simulink model "sampleModel1962_4"  (R2023a)
settings: Solver=VariableStepAuto  StartTime=0.0  StopTime=10.0  RelTol=1e-3
libraries: hdlsllib x4, simulink x3
settings Model: Creator=user1  LastModifiedBy=user1

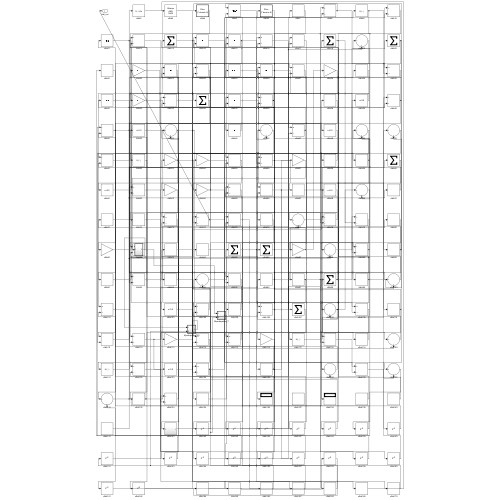
[thumbnail: Simulink's stored preview of the top-level diagram]
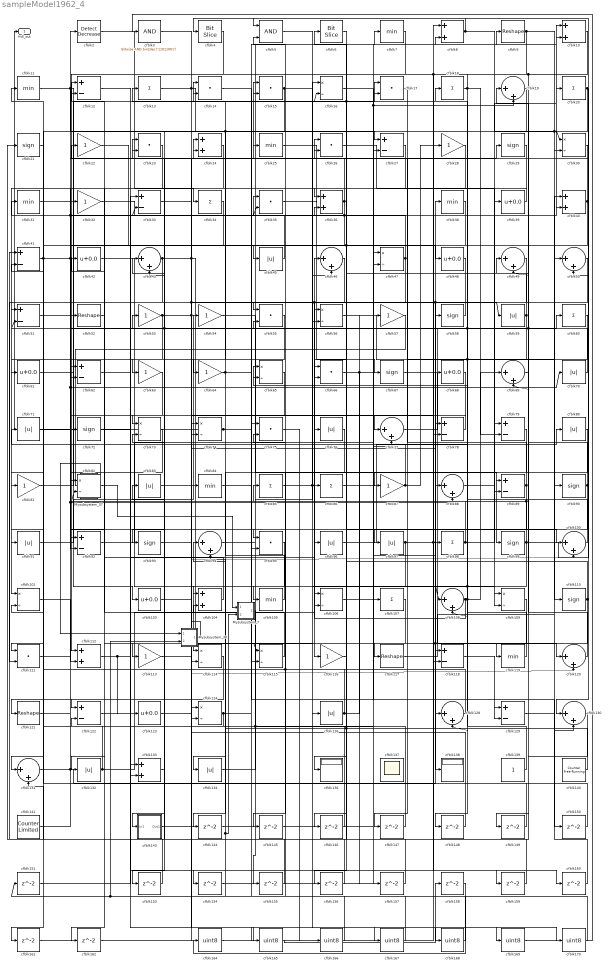
== system sampleModel1962_4 ==
  Mysubsystem_30 : Subsystem  TreatAsAtomicUnit=on  RTWFcnName=Mysubsystem_30
      settings: RTWFcnNameOpts=User specified  RTWFileNameOpts=Use function name
  Mysubsystem_37 : Subsystem  TreatAsAtomicUnit=on  RTWFcnName=Mysubsystem_37
      settings: RTWFcnNameOpts=User specified  RTWFileNameOpts=Use function name
  Mysubsystem_7 : Subsystem  TreatAsAtomicUnit=on  RTWFcnName=Mysubsystem_7
      settings: RTWFcnNameOpts=User specified  RTWFileNameOpts=Use function name
  cfblk{8,10,24,36,40,104,112,133} (8 alike) : Sum  OutDataTypeStr=uint8
  cfblk{19,43,46,49..50,69,77,88,94,100,108,120,128,130..131} (15 alike) : Sum  Inputs=|++  OutDataTypeStr=uint8
  cfblk{16,30,47,56,65,73..74,82,101,106,109,114..115,124} (14 alike) : Product  Inputs=*/  OutDataTypeStr=uint8  RndMeth=Zero  SaturateOnIntegerOverflow=on
  cfblk{39,42,48,61,68,103,123} (7 alike) : Bias  Bias=0.0  SaturateOnIntegerOverflow=off
  cfblk{7,11,25,31,38,84,105,119} (8 alike) : MinMax  OutDataTypeStr=uint8
  cfblk{13,18,20,34,60,85..86,98,107} (9 alike) : Sum  Inputs=+  OutDataTypeStr=uint8
  cfblk{21,29,58,67,72,90,93,99,110} (9 alike) : Signum
  cfblk{14..15,17,23,26,35,55,66,75,95,111} (11 alike) : DotProduct  OutDataTypeStr=uint8
  cfblk{22,28,32,53..54,57,63..64,81,87,113,116} (12 alike) : Gain  OutDataTypeStr=uint8
  cfblk{9,52,117,121} (4 alike) : Reshape
  cfblk{12,27,33,41,51,62,78..79,89,92,118,122,129} (13 alike) : Sum  Inputs=+-  OutDataTypeStr=uint8
  cfblk{45,59,70..71,76,80,83,91,96..97,126,132,134} (13 alike) : Abs  OutDataTypeStr=uint8  SaturateOnIntegerOverflow=off
  cfblk136 : Display
  cfblk137 : Scope
      settings: Floating=on
  cfblk138 : Display
  cfblk139 : Constant  OutDataTypeStr=uint8  SampleTime=-1
  cfblk140 : hdlsllib/Sources/Counter Free-Running  NumBits=16  tsamp=-1
  cfblk141 : hdlsllib/Sources/Counter Limited  uplimit=7  tsamp=-1
  cfblk143 : Subsystem
      settings: LibrarySourceBlock=|
      | hdlsllib/Ports &
      | Subsystems/Subsystem
  cfblk{144..151,153..162} (18 alike) : Delay  SampleTime=1
  cfblk{164..170} (7 alike) : DataTypeConversion  OutDataTypeStr=uint8  SaturateOnIntegerOverflow=off  RndMeth=Floor
  cfblk2 : simulink/Logic and Bit Operations/Detect Decrease  vinit=0.0  OutDataTypeStr=uint8
      settings: LibrarySourceBlock=|
      | hdlsllib/Logic and Bit
      | Operations/Detect
      | Decrease
  cfblk3 : simulink/Logic and Bit Operations/Bitwise Operator  logicop=AND  UseBitMask=on  BitMask=bin2dec('11011001')  BitMaskRealWorld=Stored Integer
      settings: LibrarySourceBlock=|
      | hdlsllib/Logic and Bit
      | Operations/Bitwise
      | Operator
  cfblk4 : hdlsllib/Logic and Bit Operations/Bit Slice  lidx=7  ridx=0
  cfblk5 : Logic  AllPortsSameDT=off  OutDataTypeStr=boolean
  cfblk6 : hdlsllib/Logic and Bit Operations/Bit Slice  lidx=7  ridx=0
  Hdl_out : Outport  OutDataTypeStr=uint8
  wires:
  cfblk134/1 -> cfblk7/1, cfblk27/2
  cfblk11/1 -> cfblk103/1, cfblk27/1
  cfblk131/1 -> cfblk38/1, cfblk55/2
  cfblk90/1 -> cfblk50/2, cfblk19/1, cfblk146/1
  cfblk42/1 -> cfblk114/1
  cfblk81/1 -> cfblk17/1
  cfblk2/1 -> cfblk34/1
  cfblk16/1 -> cfblk107/1, cfblk19/2
  cfblk98/1 -> cfblk85/1, cfblk20/1
  cfblk17/1 -> cfblk77/1
  cfblk22/1 -> cfblk45/1
  cfblk49/1 -> cfblk116/1, cfblk143/1(In1)
  cfblk50/1 -> cfblk138/1, cfblk147/1
  cfblk63/1 -> cfblk112/1
  cfblk78/1 -> cfblk73/1
  cfblk24/1 -> cfblk101/1
  cfblk4/1 -> cfblk72/1
  cfblk58/1 -> cfblk51/1
  cfblk54/1 -> cfblk99/1
  cfblk26/1 -> cfblk109/1
  cfblk64/1 -> cfblk24/1, cfblk130/2
  cfblk67/1 -> cfblk119/1
  cfblk41/1 -> cfblk48/1, cfblk95/2, cfblk131/1
  cfblk96/1 -> cfblk80/1
  cfblk38/1 -> cfblk81/1, cfblk106/1
  cfblk87/1 -> cfblk14/1, cfblk28/1
  cfblk86/1 -> cfblk89/1
  cfblk25/1 -> cfblk67/1
  cfblk45/1 -> cfblk24/2
  cfblk39/1 -> cfblk32/1
  cfblk6/1 -> cfblk136/1
  cfblk108/1 -> cfblk18/1, cfblk69/1, cfblk106/2
  cfblk84/1 -> cfblk9/1
  cfblk48/1 -> cfblk111/1
  cfblk70/1 -> cfblk12/1, cfblk43/1, cfblk49/2
  cfblk119/1 -> cfblk13/1, cfblk51/2
  cfblk92/1 -> cfblk10/1
  cfblk97/1 -> cfblk120/1, cfblk159/1, cfblk105/1
  cfblk43/1 -> cfblk126/1, cfblk78/2, cfblk111/2
  cfblk100/1 -> cfblk71/1
  cfblk115/1 -> cfblk12/2
  cfblk21/1 -> cfblk91/1
  cfblk113/1 -> cfblk29/1
  cfblk99/1 -> cfblk4/1, cfblk134/1, cfblk65/1
  cfblk61/1 -> cfblk10/2
  cfblk40/1 -> cfblk22/1, cfblk43/2
  cfblk71/1 -> cfblk62/1
  cfblk51/1 -> cfblk2/1
  cfblk83/1 -> cfblk54/1
  cfblk132/1 -> cfblk46/1, cfblk41/2
  cfblk27/1 -> cfblk62/2
  cfblk52/1 -> cfblk132/1
  cfblk74/1 -> cfblk56/1, Hdl_out/1
  cfblk139/1 -> cfblk15/1
  cfblk20/1 -> cfblk64/1, cfblk61/1, cfblk130/1
  cfblk23/1 -> cfblk52/1
  cfblk9/1 -> cfblk110/1, cfblk88/1
  cfblk106/1 -> cfblk98/1
  cfblk101/1 -> cfblk112/2
  cfblk118/1 -> cfblk129/1
  cfblk47/1 -> cfblk93/1, cfblk35/1
  cfblk18/1 -> cfblk58/1, cfblk79/2
  cfblk109/1 -> cfblk122/1
  cfblk94/1 -> cfblk16/1
  cfblk89/1 -> cfblk97/1, cfblk82/2, cfblk25/1
  cfblk53/1 -> cfblk55/1, cfblk120/2, cfblk161/1
  cfblk111/1 -> cfblk26/1, cfblk88/2
  cfblk13/1 -> cfblk47/1, cfblk56/2
  cfblk46/1 -> cfblk113/1
  cfblk121/1 -> cfblk53/1
  cfblk143/1(Out1) -> cfblk47/2
  cfblk59/1 -> cfblk108/1, cfblk128/2, cfblk31/1
  cfblk133/1 -> cfblk23/1
  cfblk32/1 -> cfblk40/2
  cfblk130/1 -> cfblk21/1
  cfblk3/1 -> cfblk170/1
  cfblk29/1 -> cfblk76/1
  cfblk104/1 -> cfblk42/1
  cfblk91/1 -> cfblk84/1
  cfblk12/1 -> cfblk100/1
  cfblk36/1 -> cfblk92/2, cfblk33/2, cfblk15/2
  cfblk60/1 -> cfblk117/1, cfblk108/2
  cfblk75/1 -> cfblk166/1
  cfblk14/1 -> cfblk129/2
  cfblk85/1 -> cfblk86/1, cfblk109/2
  cfblk15/1 -> cfblk46/2, cfblk153/1
  cfblk140/1 -> cfblk16/2, cfblk6/1, cfblk104/2
  cfblk112/1 -> cfblk96/1, cfblk123/1
  cfblk30/1 -> cfblk26/2
  cfblk110/1 -> cfblk115/1, cfblk118/1, cfblk66/2
  cfblk93/1 -> cfblk115/2
  cfblk141/1 -> cfblk60/1, cfblk70/1
  cfblk68/1 -> cfblk87/1
  cfblk95/1 -> cfblk104/1
  cfblk55/1 -> cfblk63/1
  cfblk128/1 -> cfblk11/1
  cfblk66/1 -> cfblk128/1, cfblk157/1
  cfblk120/1 -> cfblk49/1
  cfblk107/1 -> cfblk133/2
  cfblk77/1 -> cfblk39/1
  cfblk10/1 -> cfblk74/2, cfblk118/2, cfblk69/2
  cfblk105/1 -> cfblk14/2
  cfblk35/1 -> cfblk68/1
  cfblk34/1 -> cfblk82/1
  cfblk28/1 -> cfblk66/1
  cfblk33/1 -> cfblk100/2, cfblk59/1
  cfblk8/1 -> cfblk30/1, cfblk30/2, cfblk5/1
  cfblk88/1 -> cfblk79/1
  cfblk114/1 -> cfblk121/1
  cfblk79/1 -> cfblk89/2
  cfblk117/1 -> cfblk50/1
  cfblk123/1 -> cfblk78/1
  cfblk56/1 -> cfblk90/1
  cfblk126/1 -> cfblk83/1, cfblk65/2, cfblk57/1
  cfblk124/1 -> cfblk8/2, cfblk122/2
  cfblk7/1 -> cfblk36/1
  cfblk73/1 -> cfblk92/1
  cfblk31/1 -> cfblk95/1, cfblk35/2
  cfblk76/1 -> cfblk144/1
  cfblk144/1 -> cfblk94/2
  cfblk80/1 -> cfblk145/1
  cfblk145/1 -> cfblk77/2
  cfblk146/1 -> cfblk124/1
  cfblk147/1 -> cfblk73/2
  cfblk19/1 -> cfblk148/1
  cfblk148/1 -> cfblk74/1
  cfblk69/1 -> cfblk149/1
  cfblk149/1 -> cfblk101/2
  cfblk129/1 -> cfblk150/1
  cfblk150/1 -> cfblk5/2
  cfblk151/1 -> cfblk133/1
  cfblk153/1 -> cfblk41/1
  cfblk62/1 -> cfblk154/1
  cfblk154/1 -> cfblk17/2
  cfblk155/1 -> cfblk33/1
  cfblk116/1 -> cfblk156/1
  cfblk156/1 -> cfblk131/2
  cfblk157/1 -> cfblk23/2
  cfblk159/1 -> cfblk36/2
  cfblk122/1 -> cfblk160/1
  cfblk160/1 -> cfblk40/1
  cfblk161/1 -> cfblk114/2
  cfblk65/1 -> cfblk162/1
  cfblk162/1 -> cfblk8/1
  cfblk158/1 -> cfblk164/1
  cfblk103/1 -> cfblk165/1
  cfblk165/1 -> cfblk158/1
  cfblk166/1 -> Mysubsystem_7/2(In2), cfblk94/1
  cfblk5/1 -> cfblk167/1
  cfblk167/1 -> cfblk75/1
  cfblk164/1 -> cfblk168/1
  cfblk168/1 -> cfblk75/2
  cfblk72/1 -> cfblk169/1
  cfblk169/1 -> cfblk3/1
  cfblk170/1 -> cfblk151/1, Mysubsystem_30/2(In2)
  cfblk82/1 -> Mysubsystem_7/1(In1)
  Mysubsystem_7/1(Out1) -> cfblk155/1
  Mysubsystem_30/1(Out1) -> cfblk124/2
  cfblk57/1 -> Mysubsystem_37/1(In1)
  Mysubsystem_37/1(Y) -> Mysubsystem_30/1(In1)

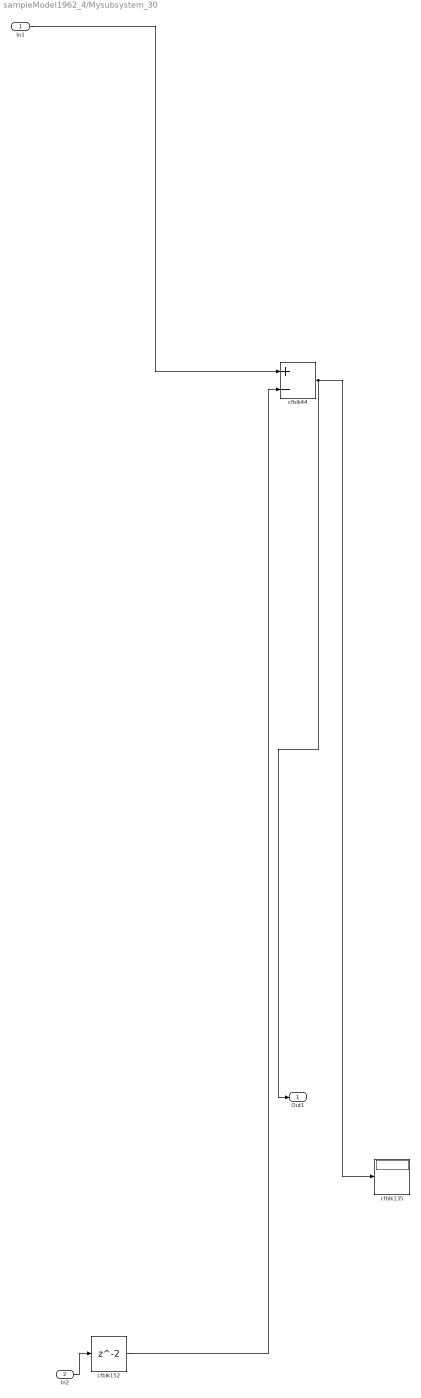
== system sampleModel1962_4/Mysubsystem_30 ==
  In1 : Inport
  In2 : Inport  Port=2
  cfblk135 : Display
  cfblk152 : Delay  SampleTime=1
  cfblk44 : Sum  Inputs=+-
  Out1 : Outport
  wires:
  In1/1 -> cfblk44/1
  cfblk152/1 -> cfblk44/2
  In2/1 -> cfblk152/1
  cfblk44/1 -> Out1/1, cfblk135/1

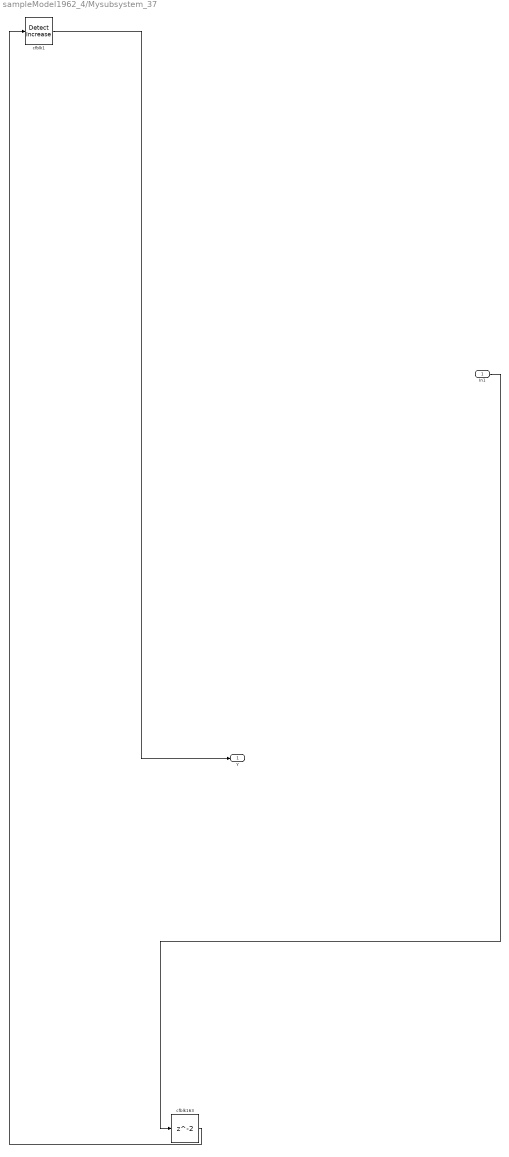
== system sampleModel1962_4/Mysubsystem_37 ==
  In1 : Inport
  cfblk1 : simulink/Logic and Bit Operations/Detect Increase  vinit=0.0  OutDataTypeStr=boolean
      settings: LibrarySourceBlock=|
      | hdlsllib/Logic and Bit
      | Operations/Detect
      | Increase
  cfblk163 : Delay  SampleTime=1
  Y : Outport
  wires:
  cfblk163/1 -> cfblk1/1
  In1/1 -> cfblk163/1
  cfblk1/1 -> Y/1

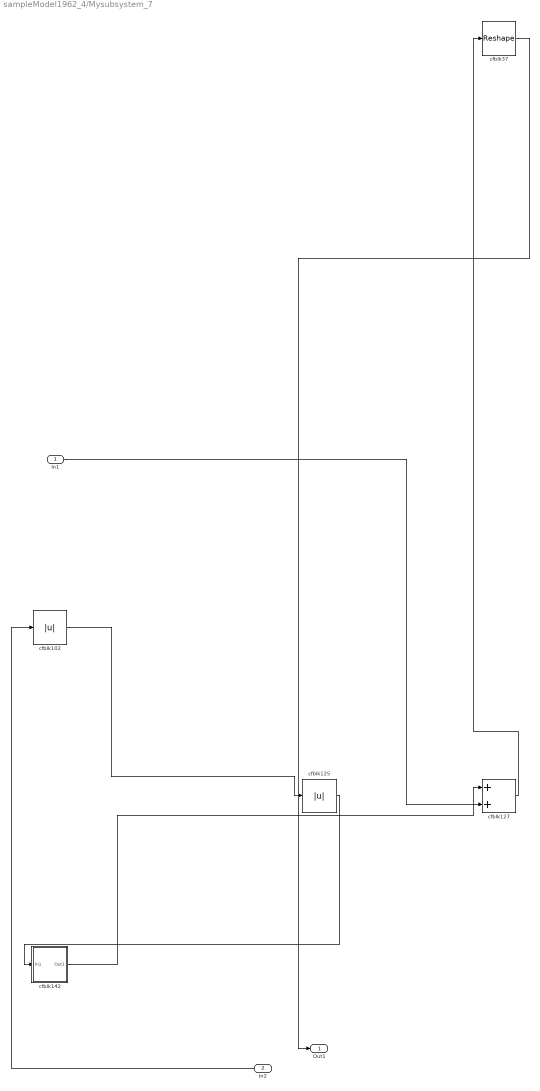
== system sampleModel1962_4/Mysubsystem_7 ==
  In1 : Inport
  In2 : Inport  Port=2
  cfblk102 : Abs  SaturateOnIntegerOverflow=off
  cfblk125 : Abs  SaturateOnIntegerOverflow=off
  cfblk127 : Sum
  cfblk142 : Subsystem
      settings: LibrarySourceBlock=|
      | hdlsllib/Ports &
      | Subsystems/Subsystem
  cfblk37 : Reshape
  Out1 : Outport
  wires:
  cfblk102/1 -> cfblk125/1
  cfblk127/1 -> cfblk37/1
  cfblk125/1 -> cfblk142/1(In1)
  cfblk37/1 -> Out1/1
  In1/1 -> cfblk127/2
  cfblk142/1(Out1) -> cfblk127/1
  In2/1 -> cfblk102/1

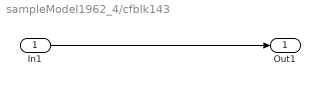
== system sampleModel1962_4/cfblk143 ==
  In1 : Inport
  Out1 : Outport
  wires:
  In1/1 -> Out1/1

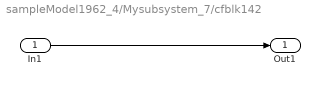
== system sampleModel1962_4/Mysubsystem_7/cfblk142 ==
  In1 : Inport
  Out1 : Outport
  wires:
  In1/1 -> Out1/1
